simulink model "lindiscrmodel_lqr_uu"  (R2019a)
settings: Solver=VariableStepAuto  StartTime=0.0  StopTime=30  RelTol=1e-3
InitFcn:
  | lindiscrmodel
values from neighbouring files (symbols this model uses):
  Ts = 0.01    [lindiscrmodel.m]
undefined symbols (not defined in the file or in its folder): Discrete, K2, linmat, Time
libraries: dspsrcs4 x2, ctrlSharedLib x1
settings Model: Creator=jessi  LastModifiedBy=jessi

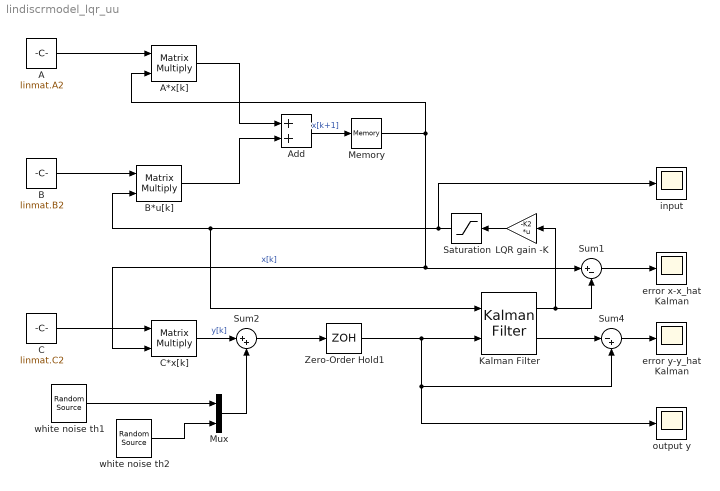
== system lindiscrmodel_lqr_uu ==
  A : Constant  Value=linmat.A2  SampleTime=Ts
  A*x[k] : Product  Multiplication=Matrix(*)
  Add : Sum
  B : Constant  Value=linmat.B2  SampleTime=Ts
  B*u[k] : Product  Multiplication=Matrix(*)
  C : Constant  Value=linmat.C2  SampleTime=Ts
  C*x[k] : Product  Multiplication=Matrix(*)
  Kalman Filter : ctrlSharedLib/Kalman Filter  TimeDomain=Discrete-Time  UseCurrentEstimator=on  ModelSource=Individual A, B, C, D matrices  ModelSourceVariable=sysd2  A=linmat.A2  B=linmat.B2  C=linmat.C2  D=linmat.D2  NumberOfStates=1  NumberOfInputs=1  NumberOfOutputs=1  InitialEstimateSource=Dialog  X0=[0.2;0;0;0]  P0=10  UseK=off  UseGH=off  NumberOfProcessNoiseInputs=1  G=1  TimeInvariantG=on  H=0  TimeInvariantH=on  Q=diag([100 100 0.01 1000])  TimeInvariantQ=on  R=0.0001  TimeInvariantR=on  N=0  TimeInvariantN=on  AddInputPort=on  AddEnablePort=off  OutputEstimatedY=on  OutputP=off  Ts=Ts
      settings: SourceProductBaseCode=CT
  LQR gain -K : Gain  Gain=-K2  Multiplication=Matrix(K*u)
  Memory : Memory  InitialCondition=[0.2;0;0;0]
  Mux : Mux  Inputs=2
  Saturation : Saturate  UpperLimit=1  LowerLimit=-1
  Sum1 : Sum  Inputs=|+-
  Sum2 : Sum  Inputs=|++
  Sum4 : Sum  Inputs=|-+
  Zero-Order Hold1 : ZeroOrderHold  SampleTime=Ts
  error x-x_hat Kalman : Scope
  error y-y_hat Kalman : Scope
  input : Scope
  output y : Scope
  white noise th1 : dspsrcs4/Random Source  SrcType=Gaussian  NormMethod=Ziggurat  CltLength=12  MinVal=0  MaxVal=1  MeanVal=0  VarVal=0.000001  RepMode=Not repeatable  rawSeed=1  IsInherit=off  SampMode=Discrete  SampTime=0.01  SampFrame=1  DataType=Double  OutComplex=Real  OutputFrames=off
  white noise th2 : dspsrcs4/Random Source  SrcType=Gaussian  NormMethod=Ziggurat  CltLength=12  MinVal=0  MaxVal=1  MeanVal=0  VarVal=0.000001  RepMode=Not repeatable  rawSeed=1  IsInherit=off  SampMode=Discrete  SampTime=0.01  SampFrame=1  DataType=Double  OutComplex=Real  OutputFrames=off
  wires:
  B/1 -> B*u[k]/1
  A/1 -> A*x[k]/1
  A*x[k]/1 -> Add/1
  B*u[k]/1 -> Add/2
  Memory/1 -> A*x[k]/2, Sum1/1, C*x[k]/2  "x[k]"
  C/1 -> C*x[k]/1
  Add/1 -> Memory/1  "x[k+1]"
  Sum1/1 -> error x-x_hat Kalman/1
  Kalman Filter/1 -> LQR gain -K/1, Sum1/2
  C*x[k]/1 -> Sum2/1  "y[k]"
  Sum4/1 -> error y-y_hat Kalman/1
  Sum2/1 -> Zero-Order Hold1/1
  Zero-Order Hold1/1 -> output y/1, Sum4/2, Kalman Filter/2
  LQR gain -K/1 -> Saturation/1
  Saturation/1 -> input/1, Kalman Filter/1, B*u[k]/2
  Kalman Filter/2 -> Sum4/1
  white noise th2/1 -> Mux/2
  white noise th1/1 -> Mux/1
  Mux/1 -> Sum2/2
